simulink model "LTI_DT_60s_sample"  (R2017a)
settings: Solver=VariableStepAuto  StartTime=0.0  StopTime=18000  RelTol=1e-3  EnableMultiTasking=on
values from neighbouring files (symbols this model uses):
  Asys = Asys_ori.*A_adj    [Asys_Creation.m]
  Bsys = zeros(no_region,no_Inputs)    [Asys_Creation.m]
  Kv_r = Kv.*SparMat    [DTContTree.m]
  L = zeros(no_region)    [Asys_Creation.m]
  no_region = numBubbles    (= 50)    [Main.m]
  root = 39    [Main.m]
  T = 60    [Main.m]
settings Model: Creator=yaqiz  LastModifiedBy=Yaqi
settings OptimizationCC: LifeSpan=inf
settings DebuggingCC: SFUnexpectedBacktrackingDiag=warning  SFNoUnconditionalDefaultTransitionDiag=warning  SFExecutionAtInitializationDiag=none
settings GRTTargetCC: TargetLangStandard=C89/C90 (ANSI)  GeneratePreprocessorConditionals=Disable all
settings ConfigComp: CovMetricSettings=dw  CovHtmlReporting=on  CovSaveCumulativeToWorkspaceVar=on  CovSaveSingleToWorkspaceVar=on  CovExternalEMLEnable=off

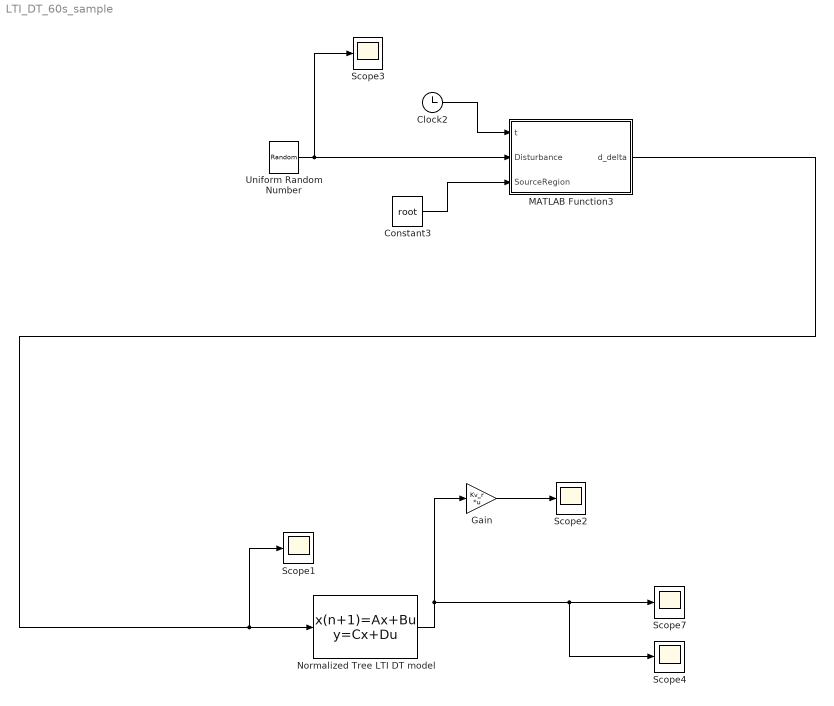
== system LTI_DT_60s_sample ==
  Clock2 : Clock
  Constant3 : Constant  Value=root
  Gain : Gain  Gain=Kv_r  Multiplication=Matrix(K*u)
  MATLAB Function3 : MATLAB Function  TreatAsAtomicUnit=on
  Normalized Tree LTI DT model : DiscreteStateSpace  A=eye(no_region)+T*L*(Asys + Bsys*Kv_r)*inv(L)  B=L*T  C=eye(no_region)  D=zeros(no_region)  X0=zeros(no_region,1)  SampleTime=60
  Scope{1..4,7} (5 alike) : Scope
  Uniform Random Number : UniformRandomNumber  SampleTime=0.1
  wires:
  Clock2/1 -> MATLAB Function3/1(t)
  Constant3/1 -> MATLAB Function3/3(SourceRegion)
  Normalized Tree LTI DT model/1 -> Gain/1, Scope4/1, Scope7/1
  Gain/1 -> Scope2/1
  MATLAB Function3/1(d_delta) -> Scope1/1, Normalized Tree LTI DT model/1
  Uniform Random Number/1 -> Scope3/1, MATLAB Function3/2(Disturbance)

== matlab function LTI_DT_60s_sample/MATLAB Function3 ==
  data: t input; Disturbance input; SourceRegion input; d_delta output size=no_region
function d_delta = fcn(t,Disturbance,SourceRegion)

% coder.varsize('d_delta', [50 1]); %n must never exceed 1024
d_delta = zeros(50,1);

 if t <= 1000000
     d_delta(SourceRegion) = Disturbance;
 end
    
end
